simulink model "ROV2"  (R2017a)
settings: Solver=VariableStepAuto  StartTime=0.0  StopTime=7  RelTol=1e-3
values from neighbouring files (symbols this model uses):
  a1 = pi/4    (= 0.785398163397)    [attitudeROV2.m]
  a2 = a1    (= 0.785398163397)    [attitudeROV2.m]
  a5 = 0    [attitudeROV2.m]
  a6 = a5    (= 0)    [attitudeROV2.m]
  Ap = 0.8337    [attitudeROV2.m]
  B = 1.82*9.8    (= 17.836)    [attitudeROV2.m]
  Bq = 0.7987    [attitudeROV2.m]
  Cr = 1.1250    (= 1.125)    [attitudeROV2.m]
  In = [0.05;0.04;0;pi/4;pi/3;pi/6]    [attitudeROV2.m]
  Kp = -0.8842    [attitudeROV2.m]
  Kpp = -0.6682    [attitudeROV2.m]
  lx1 = 0.19    [attitudeROV2.m]
  lx2 = 0.19    [attitudeROV2.m]
  lx5 = 0.17    [attitudeROV2.m]
  lx6 = -0.17    [attitudeROV2.m]
  ly1 = 0.11    [attitudeROV2.m]
  ly2 = 0.11    [attitudeROV2.m]
  ly3 = 0.11    [attitudeROV2.m]
  ly4 = 0.11    [attitudeROV2.m]
  ly5 = 0.11    [attitudeROV2.m]
  ly6 = 0.11    [attitudeROV2.m]
  lz = 0.19    [attitudeROV2.m]
  m = 6.621    [attitudeROV2.m]
  Mq = -0.8547    [attitudeROV2.m]
  Mqq = -0.3354    [attitudeROV2.m]
  Nr = -1.0280    (= -1.028)    [attitudeROV2.m]
  Nrr = -1.0249    [attitudeROV2.m]
  Tgadd = [0,0,-0.25,0.5,0.25,0 ... (first row only)    [attitudeROV2.m]
  Tn = inv(T)    [attitudeROV2.m]
  zB = -0.042    [attitudeROV2.m]
libraries: simulink x3, aerolibutil x1, sharedutil x1
settings Model: Creator=52958  LastModifiedBy=admin

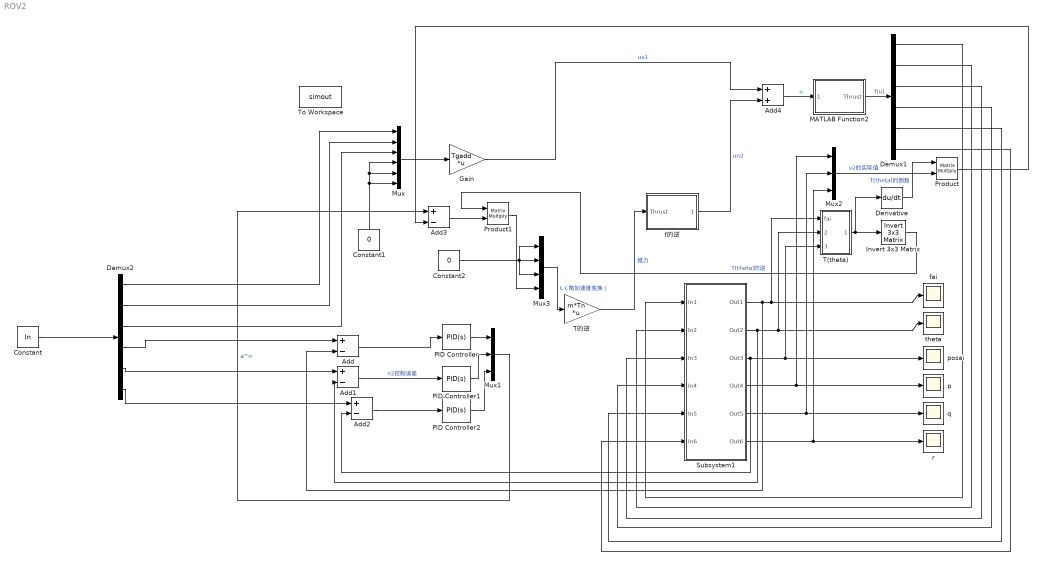
== system ROV2 ==
  Add{,1..3} (4 alike) : Sum  Inputs=+-
  Add4 : Sum
  Constant : Constant  Value=In
  Constant1 : Constant  Value=0
  Constant2 : Constant  Value=0
  Demux1 : Demux  Outputs=6
  Demux2 : Demux  Outputs=6
  Derivative : Derivative
  Gain : Gain  Gain=Tgadd  Multiplication=Matrix(K*u)
  Invert 3x3 Matrix : aerolibutil/Invert  3x3 Matrix
  MATLAB Function2 : MATLAB Function  TreatAsAtomicUnit=on
  Mux : Mux  Inputs=6
  Mux1 : Mux  Inputs=3
  Mux2 : Mux  Inputs=3
  Mux3 : Mux
  PID Controller : simulink/Continuous/PID Controller  Controller=PID  TimeDomain=Continuous-time  SampleTime=-1  IntegratorMethod=Forward Euler  FilterMethod=Forward Euler  Form=Parallel  UseFilter=on  ControllerParametersSource=internal  P=2  I=0.1  D=0.1  N=100  InitialConditionSource=internal  InitialConditionForIntegrator=0  InitialConditionForFilter=0  ExternalReset=none  LimitOutput=off  UpperSaturationLimit=inf  LowerSaturationLimit=-inf  LinearizeAsGain=on  AntiWindupMode=none  Kb=1  TrackingMode=off  Kt=1  PParamMin=[]  PParamMax=[]  IParamMin=[]  IParamMax=[]  DParamMin=[]  DParamMax=[]  NParamMin=[]  NParamMax=[]  KbParamMin=[]  KbParamMax=[]  KtParamMin=[]  KtParamMax=[]  POutMin=[]  POutMax=[]  IOutMin=[]  IOutMax=[]  DOutMin=[]  DOutMax=[]  NOutMin=[]  NOutMax=[]  KbOutMin=[]  KbOutMax=[]  KtOutMin=[]  KtOutMax=[]  IntegratorOutMin=[]  IntegratorOutMax=[]  FilterOutMin=[]  FilterOutMax=[]  SumOutMin=[]  SumOutMax=[]  SumI1OutMin=[]  SumI1OutMax=[]  SumI2OutMin=[]  SumI2OutMax=[]  SumI3OutMin=[]  SumI3OutMax=[]  SumDOutMin=[]  SumDOutMax=[]  SaturationOutMin=[]  SaturationOutMax=[]  IntegratorContinuousStateAttributes=''  IntegratorStateMustResolveToSignalObject=off  IntegratorRTWStateStorageClass=Auto  FilterContinuousStateAttributes=''  FilterStateMustResolveToSignalObject=off  FilterRTWStateStorageClass=Auto  DifferentiatorICPrevScaledInput=0  DifferentiatorOutMin=[]  DifferentiatorOutMax=[]  InitialConditionSetting=State (most efficient)
  PID Controller1 : simulink/Continuous/PID Controller  Controller=PID  TimeDomain=Continuous-time  SampleTime=-1  IntegratorMethod=Forward Euler  FilterMethod=Forward Euler  Form=Parallel  UseFilter=on  ControllerParametersSource=internal  P=2.7  I=0.1  D=0.1  N=100  InitialConditionSource=internal  InitialConditionForIntegrator=0  InitialConditionForFilter=0  ExternalReset=none  LimitOutput=off  UpperSaturationLimit=inf  LowerSaturationLimit=-inf  LinearizeAsGain=on  AntiWindupMode=none  Kb=1  TrackingMode=off  Kt=1  PParamMin=[]  PParamMax=[]  IParamMin=[]  IParamMax=[]  DParamMin=[]  DParamMax=[]  NParamMin=[]  NParamMax=[]  KbParamMin=[]  KbParamMax=[]  KtParamMin=[]  KtParamMax=[]  POutMin=[]  POutMax=[]  IOutMin=[]  IOutMax=[]  DOutMin=[]  DOutMax=[]  NOutMin=[]  NOutMax=[]  KbOutMin=[]  KbOutMax=[]  KtOutMin=[]  KtOutMax=[]  IntegratorOutMin=[]  IntegratorOutMax=[]  FilterOutMin=[]  FilterOutMax=[]  SumOutMin=[]  SumOutMax=[]  SumI1OutMin=[]  SumI1OutMax=[]  SumI2OutMin=[]  SumI2OutMax=[]  SumI3OutMin=[]  SumI3OutMax=[]  SumDOutMin=[]  SumDOutMax=[]  SaturationOutMin=[]  SaturationOutMax=[]  IntegratorContinuousStateAttributes=''  IntegratorStateMustResolveToSignalObject=off  IntegratorRTWStateStorageClass=Auto  FilterContinuousStateAttributes=''  FilterStateMustResolveToSignalObject=off  FilterRTWStateStorageClass=Auto  DifferentiatorICPrevScaledInput=0  DifferentiatorOutMin=[]  DifferentiatorOutMax=[]  InitialConditionSetting=State (most efficient)
  PID Controller2 : simulink/Continuous/PID Controller  Controller=PID  TimeDomain=Continuous-time  SampleTime=-1  IntegratorMethod=Forward Euler  FilterMethod=Forward Euler  Form=Parallel  UseFilter=on  ControllerParametersSource=internal  P=0.7  I=0.1  D=0.1  N=100  InitialConditionSource=internal  InitialConditionForIntegrator=0  InitialConditionForFilter=0  ExternalReset=none  LimitOutput=off  UpperSaturationLimit=inf  LowerSaturationLimit=-inf  LinearizeAsGain=on  AntiWindupMode=none  Kb=1  TrackingMode=off  Kt=1  PParamMin=[]  PParamMax=[]  IParamMin=[]  IParamMax=[]  DParamMin=[]  DParamMax=[]  NParamMin=[]  NParamMax=[]  KbParamMin=[]  KbParamMax=[]  KtParamMin=[]  KtParamMax=[]  POutMin=[]  POutMax=[]  IOutMin=[]  IOutMax=[]  DOutMin=[]  DOutMax=[]  NOutMin=[]  NOutMax=[]  KbOutMin=[]  KbOutMax=[]  KtOutMin=[]  KtOutMax=[]  IntegratorOutMin=[]  IntegratorOutMax=[]  FilterOutMin=[]  FilterOutMax=[]  SumOutMin=[]  SumOutMax=[]  SumI1OutMin=[]  SumI1OutMax=[]  SumI2OutMin=[]  SumI2OutMax=[]  SumI3OutMin=[]  SumI3OutMax=[]  SumDOutMin=[]  SumDOutMax=[]  SaturationOutMin=[]  SaturationOutMax=[]  IntegratorContinuousStateAttributes=''  IntegratorStateMustResolveToSignalObject=off  IntegratorRTWStateStorageClass=Auto  FilterContinuousStateAttributes=''  FilterStateMustResolveToSignalObject=off  FilterRTWStateStorageClass=Auto  DifferentiatorICPrevScaledInput=0  DifferentiatorOutMin=[]  DifferentiatorOutMax=[]  InitialConditionSetting=State (most efficient)
  Product : Product  Multiplication=Matrix(*)
  Product1 : Product  Multiplication=Matrix(*)
  Subsystem1 : Subsystem
  T(theta) : Subsystem
  To Workspace : ToWorkspace  VariableName=simout  SaveFormat=Timeseries  SampleTime=-1
  T的逆 : Gain  Gain=m*Tn  Multiplication=Matrix(K*u)
  fai : Scope
  f的逆 : MATLAB Function  TreatAsAtomicUnit=on
  p : Scope
  posai : Scope
  q : Scope
  r : Scope
  theta : Scope
  wires:
  Demux2/4 -> Add/1
  Demux2/6 -> Add2/1
  MATLAB Function2/1(Thrust) -> Demux1/1  "f(u)"
  f的逆/1(Amount) -> Add4/2  "un2"
  Constant/1 -> Demux2/1
  Product1/1 -> Mux3/4
  Subsystem1/4("Out4 ") -> p/1, Mux2/1
  Demux1/2 -> Subsystem1/2(In2)
  Constant2/1 -> Mux3/1, Mux3/3, Mux3/2
  Demux1/3 -> Subsystem1/3(In3)
  Demux1/5 -> Subsystem1/5(In5)
  Invert 3x3 Matrix/1 -> Product1/1  "T(theta)的逆"
  Demux2/2 -> Mux/2
  PID Controller2/1 -> Mux1/3
  PID Controller/1 -> Mux1/1
  Derivative/1 -> Product/1  "T(theta)的倒数"
  Subsystem1/6(Out6) -> r/1, Mux2/3
  Mux3/1 -> T的逆/1  "L（角加速度变换）"
  Add3/1 -> Product1/2
  Gain/1 -> Add4/1  "uv1"
  Mux2/1 -> Product/2  "v2的实际值"
  Add4/1 -> MATLAB Function2/1(Amount)  "u"
  T的逆/1 -> f的逆/1(Thrust)  "推力"
  Add1/1 -> PID Controller1/1  "n2控制误差"
  Add2/1 -> PID Controller2/1
  Constant1/1 -> Mux/6, Mux/5, Mux/4
  Subsystem1/3(Out3) -> Add2/2, posai/1, T(theta)/3(posai)
  Product/1 -> Add3/2
  Subsystem1/5(Out5) -> q/1, Mux2/2
  Demux2/5 -> Add1/1
  Demux2/1 -> Mux/1
  Demux1/4 -> Subsystem1/4(In4)
  T(theta)/1(Out1) -> Derivative/1, Invert 3x3 Matrix/1
  Mux1/1 -> Add3/1  "a^n"
  Subsystem1/1("Out1 ") -> T(theta)/1(fai), fai/1, Add/2
  Demux1/6 -> Subsystem1/6(In6)
  Mux/1 -> Gain/1
  Demux2/3 -> Mux/3
  PID Controller1/1 -> Mux1/2
  Demux1/1 -> Subsystem1/1(In1)
  Add/1 -> PID Controller/1
  Subsystem1/2(Out2) -> T(theta)/2(ceta), theta/1, Add1/2

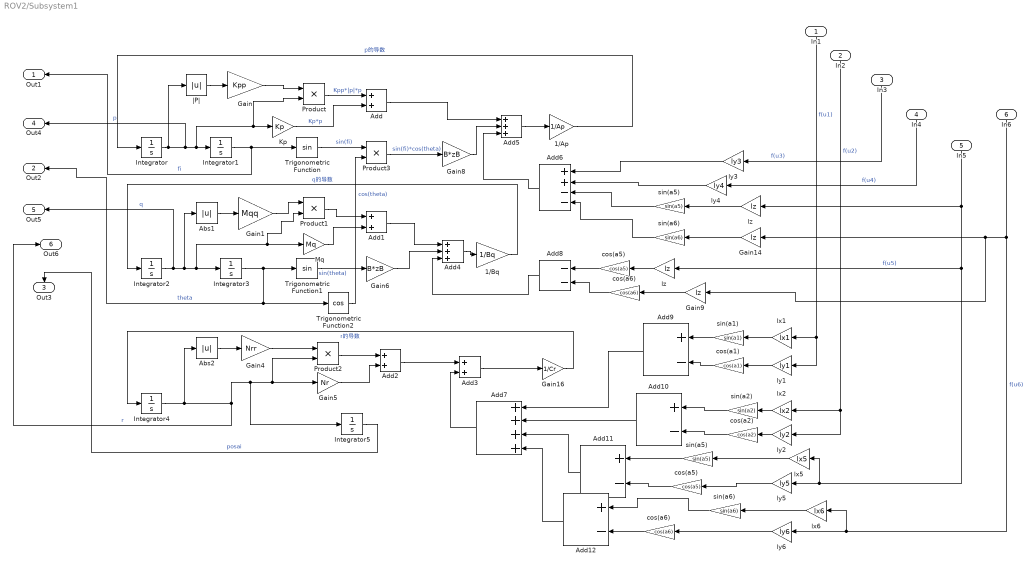
== system ROV2/Subsystem1 ==
  In1 : Inport
  In2 : Inport  Port=2
  In3 : Inport  Port=3
  In4 : Inport  Port=4
  In5 : Inport  Port=5
  In6 : Inport  Port=6
  1/Ap : Gain  Gain=1/Ap
  1/Bq : Gain  Gain=1/Bq
  Abs1 : Abs
  Abs2 : Abs
  Add{,1..3} (4 alike) : Sum
  Add{9..12} (4 alike) : Sum  Inputs=+-
  Add4 : Sum  Inputs=+++
  Add5 : Sum  Inputs=+++
  Add6 : Sum  Inputs=++--
  Add7 : Sum  Inputs=++++
  Add8 : Sum  Inputs=--
  Gain : Gain  Gain=Kpp
  Gain1 : Gain  Gain=Mqq
  Gain14 : Gain  Gain=lz
  Gain16 : Gain  Gain=1/Cr
  Gain4 : Gain  Gain=Nrr
  Gain5 : Gain  Gain=Nr
  Gain6 : Gain  Gain=B*zB
  Gain8 : Gain  Gain=B*zB
  Gain9 : Gain  Gain=lz
  Integrator{,1..5} (6 alike) : Integrator
  Kp : Gain  Gain=Kp
  Mq : Gain  Gain=Mq
  Product{,1..3} (4 alike) : Product
  Trigonometric Function : Trigonometry
  Trigonometric Function1 : Trigonometry
  Trigonometric Function2 : Trigonometry  Operator=cos
  cos(a1) : Gain  Gain=cos(a1)
  cos(a2) : Gain  Gain=cos(a2)
  cos(a5) : Gain  Gain=cos(a5)
  "cos(a5) " : Gain  Gain=cos(a5)
  cos(a6) : Gain  Gain=cos(a6)
  "cos(a6) " : Gain  Gain=cos(a6)
  lx1 : Gain  Gain=lx1
  lx2 : Gain  Gain=lx2
  lx5 : Gain  Gain=lx5
  "lx6 " : Gain  Gain=lx6
  ly1 : Gain  Gain=ly1
  ly2 : Gain  Gain=ly2
  ly3 : Gain  Gain=ly3
  ly4 : Gain  Gain=ly4
  ly5 : Gain  Gain=ly5
  ly6 : Gain  Gain=ly6
  lz : Gain  Gain=lz
  "lz " : Gain  Gain=lz
  sin(a1) : Gain  Gain=sin(a1)
  sin(a2) : Gain  Gain=sin(a2)
  sin(a5) : Gain  Gain=sin(a5)
  "sin(a5) " : Gain  Gain=sin(a5)
  sin(a6) : Gain  Gain=sin(a6)
  "sin(a6) " : Gain  Gain=sin(a6)
  |P| : Abs
  "Out1 " : Outport
  Out2 : Outport  Port=2
  Out3 : Outport  Port=3
  "Out4 " : Outport  Port=4
  Out5 : Outport  Port=5
  Out6 : Outport  Port=6
  wires:
  In6/1 -> "lx6 "/1, ly6/1, Gain9/1, Gain14/1  "f(u6)"
  Add8/1 -> Add4/3
  In5/1 -> "lz "/1, lx5/1, ly5/1, lz/1  "f(u5)"
  In3/1 -> ly3/1  "f(u3)"
  Integrator5/1 -> Out3/1  "posai"
  Add7/1 -> Add3/2
  Integrator/1 -> Kp/1, Product/2, Integrator1/1, "Out4 "/1, |P|/1  "p"
  Product/1 -> Add/1  "Kpp*|p|*p"
  Product1/1 -> Add1/1
  Gain1/1 -> Product1/1
  Add/1 -> Add5/1
  Integrator1/1 -> "Out1 "/1, Trigonometric Function/1  "fi"
  Kp/1 -> Add/2  "Kp*p"
  Product2/1 -> Add2/1
  Gain4/1 -> Product2/1
  Gain5/1 -> Add2/2
  Abs2/1 -> Gain4/1
  Integrator4/1 -> Abs2/1, Gain5/1, Product2/2, Integrator5/1, Out6/1  "r"
  Add2/1 -> Add3/1
  1/Bq/1 -> Integrator2/1  "q的导数"
  Gain16/1 -> Integrator4/1  "r的导数"
  |P|/1 -> Gain/1
  Add4/1 -> 1/Bq/1
  Gain8/1 -> Add5/2
  Add1/1 -> Add4/1
  Add6/1 -> Add5/3
  Mq/1 -> Add1/2
  Gain6/1 -> Add4/2
  Abs1/1 -> Gain1/1
  Integrator2/1 -> Product1/2, Mq/1, Integrator3/1, Abs1/1, Out5/1  "q"
  Integrator3/1 -> Trigonometric Function1/1, Trigonometric Function2/1, Out2/1  "theta"
  Trigonometric Function1/1 -> Gain6/1  "sin(theta)"
  Trigonometric Function/1 -> Product3/1  "sin(fi)"
  Trigonometric Function2/1 -> Product3/2  "cos(theta)"
  Product3/1 -> Gain8/1  "sin(fi)*cos(theta)"
  1/Ap/1 -> Integrator/1  "p的导数"
  Add3/1 -> Gain16/1
  Add5/1 -> 1/Ap/1
  Gain/1 -> Product/1
  In2/1 -> lx2/1, ly2/1  "f(u2)"
  In4/1 -> ly4/1  "f(u4)"
  In1/1 -> ly1/1, lx1/1  "f(u1)"
  Gain14/1 -> sin(a6)/1
  ly3/1 -> Add6/1
  ly4/1 -> Add6/2
  "lz "/1 -> sin(a5)/1
  sin(a5)/1 -> Add6/3
  sin(a6)/1 -> Add6/4
  lz/1 -> cos(a5)/1
  cos(a5)/1 -> Add8/1
  Gain9/1 -> cos(a6)/1
  cos(a6)/1 -> Add8/2
  lx1/1 -> sin(a1)/1
  sin(a1)/1 -> Add9/1
  ly1/1 -> cos(a1)/1
  cos(a1)/1 -> Add9/2
  Add9/1 -> Add7/1
  Add10/1 -> Add7/2
  sin(a2)/1 -> Add10/1
  cos(a2)/1 -> Add10/2
  lx2/1 -> sin(a2)/1
  ly2/1 -> cos(a2)/1
  ly5/1 -> "cos(a5) "/1
  ly6/1 -> "cos(a6) "/1
  "cos(a5) "/1 -> Add11/2
  Add11/1 -> Add7/3
  Add12/1 -> Add7/4
  "cos(a6) "/1 -> Add12/2
  lx5/1 -> "sin(a5) "/1
  "sin(a5) "/1 -> Add11/1
  "sin(a6) "/1 -> Add12/1
  "lx6 "/1 -> "sin(a6) "/1

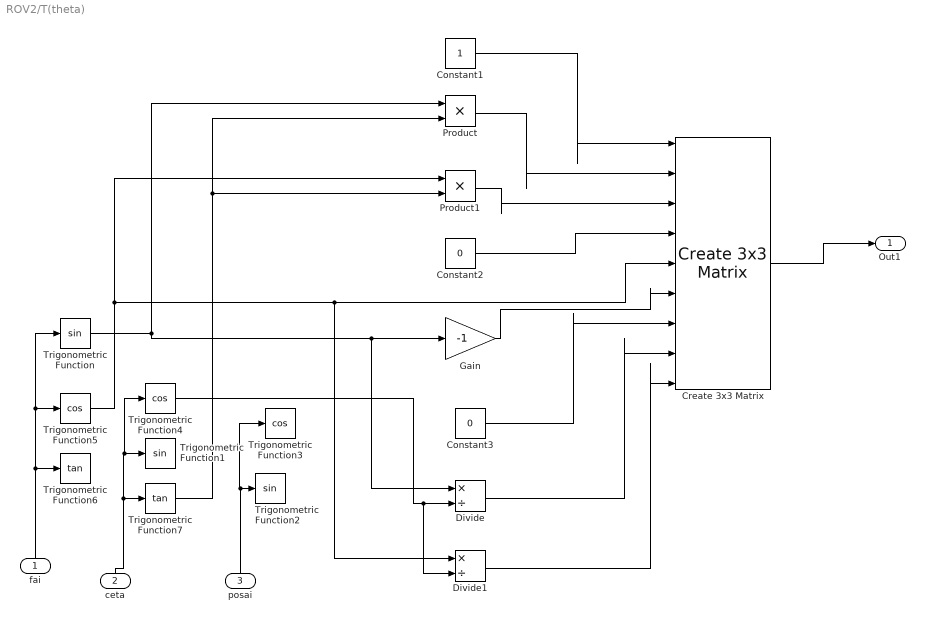
== system ROV2/T(theta) ==
  fai : Inport
  ceta : Inport  Port=2
  posai : Inport  Port=3
  Constant1 : Constant
  Constant2 : Constant  Value=0
  Constant3 : Constant  Value=0
  Create 3x3 Matrix : sharedutil/Create 3x3 Matrix
  Divide : Product  Inputs=*/
  Divide1 : Product  Inputs=*/
  Gain : Gain  Gain=-1
  Product : Product
  Product1 : Product
  Trigonometric Function : Trigonometry
  Trigonometric Function1 : Trigonometry
  Trigonometric Function2 : Trigonometry
  Trigonometric Function3 : Trigonometry  Operator=cos
  Trigonometric Function4 : Trigonometry  Operator=cos
  Trigonometric Function5 : Trigonometry  Operator=cos
  Trigonometric Function6 : Trigonometry  Operator=tan
  Trigonometric Function7 : Trigonometry  Operator=tan
  Out1 : Outport
  wires:
  posai/1 -> Trigonometric Function3/1, Trigonometric Function2/1
  fai/1 -> Trigonometric Function5/1, Trigonometric Function/1, Trigonometric Function6/1
  ceta/1 -> Trigonometric Function1/1, Trigonometric Function4/1, Trigonometric Function7/1
  Trigonometric Function7/1 -> Product1/2, Product/2
  Trigonometric Function/1 -> Divide/1, Gain/1, Product/1
  Trigonometric Function5/1 -> Create 3x3 Matrix/5, Divide1/1, Product1/1
  Trigonometric Function4/1 -> Divide1/2, Divide/2
  Constant1/1 -> Create 3x3 Matrix/1
  Product/1 -> Create 3x3 Matrix/2
  Product1/1 -> Create 3x3 Matrix/3
  Constant2/1 -> Create 3x3 Matrix/4
  Gain/1 -> Create 3x3 Matrix/6
  Constant3/1 -> Create 3x3 Matrix/7
  Divide/1 -> Create 3x3 Matrix/8
  Divide1/1 -> Create 3x3 Matrix/9
  Create 3x3 Matrix/1 -> Out1/1

== matlab function ROV2/f的逆 ==
  data: Amount output size=6; Thrust input size=6

function Amount = fcn(Thrust)
 
Amount = 0.035228317146663*Thrust + 1.41988787470481e-8*Thrust.*Thrust.*Thrust.*Thrust.*Thrust -0.0249641186721528 - 2.95262553414835e-12*Thrust.*Thrust.*Thrust.*Thrust.*Thrust.*Thrust.*Thrust - 2.28198208444611e-5*Thrust.*Thrust.*Thrust - 2.31478397188569e-5*Thrust.*Thrust;

== matlab function ROV2/MATLAB Function2 ==
  data: Amount input; Thrust output

function Thrust=fcn(Amount)
 
Thrust = 0.376932138847166 + 17.2963443077659*Amount + 97.9534845412688*Amount.*Amount.*Amount+ 61.2434082561376*Amount.*Amount.*Amount.*Amount.*Amount.*Amount.*Amount+ 3.9318327134905*Amount.*Amount - 130.236501915663*Amount.*Amount.*Amount.*Amount.*Amount;
